simulink model "R3GDL"  (Simulink 9.0)
settings: Solver=ode45  StartTime=0.0  StopTime=Tsim  MaxStep=1e-3  RelTol=1e-3  EnableMultiTasking=on
values from neighbouring files (symbols this model uses):
  A_a = [5  4.5   2]    [MinimosCuadrados.m]    (also in graficas_id.m)
  A_b = 0*[2 1.15 0.0]    [MinimosCuadrados.m]    (also in graficas_id.m)
  Icc = [0 1 0.5]    [MinimosCuadrados.m]    (also in graficas_id.m)
  R1 = 50    [MinimosCuadrados.m]    (also in ModeloDinamicoEstimado_GXX.m = 1; Reduccion.m)
  R2 = 30    [MinimosCuadrados.m]    (also in ModeloDinamicoEstimado_GXX.m = 1; Reduccion.m)
  R3 = 15    [MinimosCuadrados.m]    (also in ModeloDinamicoEstimado_GXX.m = 1; Reduccion.m)
  tau = 7    [MinimosCuadrados.m]    (also in graficas_id.m)
  Ts = 1e-3    (= 0.001)    [MinimosCuadrados.m]    (also in graficas_id.m)
  w_a = [0.5 0.5 0.5]    [MinimosCuadrados.m]    (also in graficas_id.m)
  w_b = [2.5 2.5 1.5]    [MinimosCuadrados.m]    (also in graficas_id.m)
settings Model: Creator=mortega  LastModifiedBy=Raúl  ExtModeTrigMode=oneshot  ExtModeArmWhenConnect=off
settings DataIOCC: SignalLoggingSaveFormat=ModelDataLogs
settings OptimizationCC: BlockReduction=off  BooleanDataType=off  ExpressionDepthLimit=2147483647  InitFltsAndDblsToZero=on
settings DebuggingCC: SaveWithParameterizedLinksMsg=none  SignalResolutionControl=TryResolveAllWithWarning  MultiTaskDSMMsg=warning  MultiTaskCondExecSysMsg=none  FcnCallInpInsideContextMsg=warning  StateNameClashWarn=warning  StrictBusMsg=None
settings HardwareCC: TargetUnknown=on
settings GRTTargetCC: TargetFcnLib=ansi_tfl_tmw.mat  CombineOutputUpdateFcns=off  GRTInterface=on

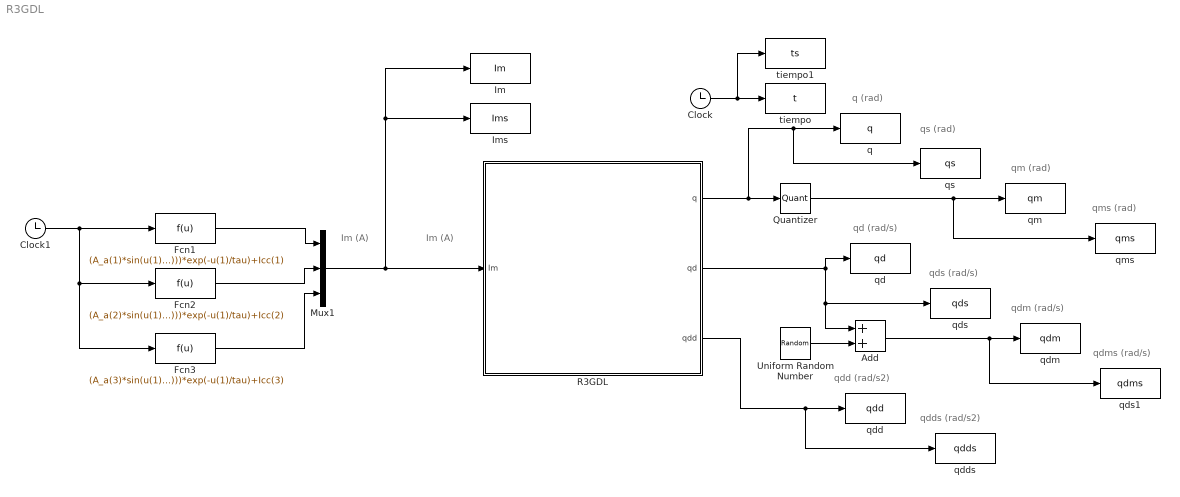
== system R3GDL ==
  note: Im (A)
  note: q (rad)
  note: qd (rad/s)
  note: qdd (rad/s2)
  note: qs (rad)
  note: qds (rad/s)
  note: qdds (rad/s2)
  note: qm (rad)
  note: qms (rad)
  note: qdm (rad/s)
  note: qdms (rad/s)
  note: Im (A)
  Add : Sum
  Clock : Clock
  Clock1 : Clock
  Fcn1 : Fcn  Expr=(A_a(1)*sin(u(1)*2*pi*w_a(1)) +A_b(1)*sin(u(1)*2*pi*w_b(1)))*exp(-u(1)/tau)+Icc(1)
  Fcn2 : Fcn  Expr=(A_a(2)*sin(u(1)*2*pi*w_a(2)) +A_b(2)*sin(u(1)*2*pi*w_b(2)))*exp(-u(1)/tau)+Icc(2)
  Fcn3 : Fcn  Expr=(A_a(3)*sin(u(1)*2*pi*w_a(3)) +A_b(3)*sin(u(1)*2*pi*w_b(3)))*exp(-u(1)/tau)+Icc(3)
  Im : ToWorkspace  VariableName=Im  SampleTime=-1
  Ims : ToWorkspace  VariableName=Ims  SampleTime=Ts
  Mux1 : Mux  Inputs=3
  Quantizer : Quantizer  QuantizationInterval=2*pi/512./[50 30 15]
  R3GDL : Subsystem  mask(Control y Programación de Robots (4 GIERM)){NGrupo=3, q1_ini=0, q2_ini=0, q3_ini=0, Bl_q1=off, Bl_q2=off, Bl_q3=off, AccionamientoDirecto=off}
      mask prompts: NGrupo "Nº de GRUPO"; q1_ini "q1 inicial  (rad)"; q2_ini "q2 inicial (rad)"; q3_ini "q3_inicial (rad)"; Bl_q1 "Bloqueo q1"; Bl_q2 "Bloqueo q2"; Bl_q3 "Bloqueo q3"; AccionamientoDirecto "Accionamiento directo"
      mask help: Robot de 3 grados de libertad RRR
      mask Display:
      | image(imread('R3GDL_RRR.JPG'));
      | port_label('output', 1, 'q');
      | port_label('output', 2, 'qd');
      | port_label('output', 3, 'qdd');
      | port_label('input', 1, 'Im')
  Uniform Random Number : UniformRandomNumber  Minimum="-0.05*[1 1 1]     %-1500*2*pi/60./[R1 R2 R3]*0.01"  Maximum="0.05*[1 1 1]     %1500*2*pi/60./[R1 R2 R3]*0.01"  SampleTime=Ts/10
  q : ToWorkspace  VariableName=q  SampleTime=-1
  qd : ToWorkspace  VariableName=qd  SampleTime=-1
  qdd : ToWorkspace  VariableName=qdd  SampleTime=-1
  qdds : ToWorkspace  VariableName=qdds  SampleTime=Ts
  qdm : ToWorkspace  VariableName=qdm  SampleTime=-1
  qds : ToWorkspace  VariableName=qds  SampleTime=Ts
  qds1 : ToWorkspace  VariableName=qdms  SampleTime=Ts
  qm : ToWorkspace  VariableName=qm  SampleTime=-1
  qms : ToWorkspace  VariableName=qms  SampleTime=Ts
  qs : ToWorkspace  VariableName=qs  SampleTime=Ts
  tiempo : ToWorkspace  VariableName=t  SampleTime=-1
  tiempo1 : ToWorkspace  VariableName=ts  SampleTime=Ts
  wires:
  Clock/1 -> tiempo1/1, tiempo/1
  Add/1 -> qdm/1, qds1/1
  Uniform Random Number/1 -> Add/2
  Quantizer/1 -> qm/1, qms/1
  R3GDL/3(qdd) -> qdd/1, qdds/1
  R3GDL/2(qd) -> qds/1, Add/1, qd/1
  R3GDL/1(q) -> Quantizer/1, q/1, qs/1
  Mux1/1 -> Ims/1, Im/1, R3GDL/1(Im)
  Clock1/1 -> Fcn3/1, Fcn2/1, Fcn1/1
  Fcn2/1 -> Mux1/2
  Fcn1/1 -> Mux1/1
  Fcn3/1 -> Mux1/3

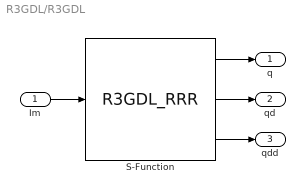
== system R3GDL/R3GDL ==
  Im : Inport
  S-Function : S-Function  FunctionName=R3GDL_RRR  Parameters=[q1_ini; q2_ini; q3_ini]; [Bl_q1; Bl_q2; Bl_q3]; AccionamientoDirecto; NGrupo  SFunctionDeploymentMode=off  EnableBusSupport=off
  q : Outport
  qd : Outport  Port=2
  qdd : Outport  Port=3
  wires:
  Im/1 -> S-Function/1
  S-Function/1 -> q/1
  S-Function/2 -> qd/1
  S-Function/3 -> qdd/1
